simulink model "tb_adc_5g_spi_sys"  (Simulink 7.0)
settings: Solver=ode45  StartTime=0.0  StopTime=2000  RelTol=1e-3
libraries: xbsIndex_r4 x446, simulink x28, xps_library x12, dspsigops x12, xbsReplacements_r4 x4, casper_library x2
(part 1 of 5)
settings Model: Creator=user  LastModifiedBy=homin
settings DebuggingCC: SaveWithParameterizedLinksMsg=none

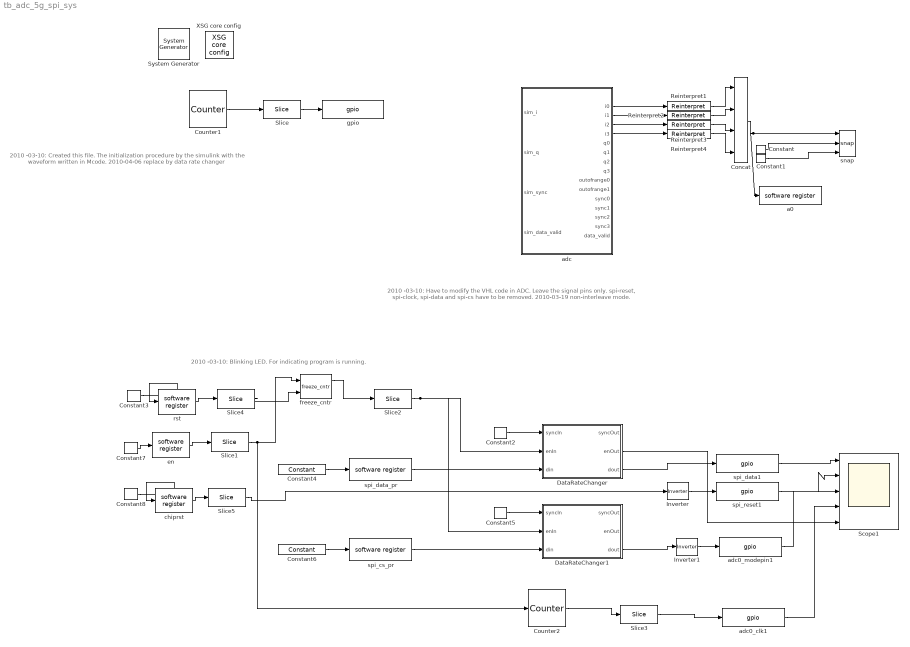
== system tb_adc_5g_spi_sys ==
  note: 2010 -03-10:
      | Created this file. The initialization procedure by the simulink with
      | the waveform written in Mcode.
      | 2010-04-06
      | replace by data rate changer
  note: 2010 -03-10:
      | Blinking LED. For indicating program is running.
  note: 2010 -03-10:
      | Have to modify the VHL code in ADC. Leave the signal pins only. spi-reset,
      | spi-clock, spi-data and spi-cs have to be removed.
      | 2010-03-19
      | non-interleave mode.
  " System Generator" : xbsIndex_r4/ System Generator  Tag=genX  SystemSampleTime=-1  xilinxfamily=virtex5  part=xc5vsx95t  speed=-1  package=ff1136  synthesis_tool=XST  clock_wrapper=Clock Enables  directory=./tb_adc_5g_spi_rw/sysgen  testbench=off  simulink_period=1  sysclk_period=5  dcm_input_clock_period=100  incr_netlist=off  trim_vbits=Everywhere in SubSystem  dbl_ovrd=According to Block Masks  core_generation=According to Block Masks  run_coregen=off  deprecated_control=off  eval_field=0  block_type=sysgen
      settings: block_version=10.1.3
  Concat : xbsIndex_r4/Concat  num_inputs=4  dbl_ovrd=off  block_type=concat
      settings: block_version=10.1.3
  Constant : xbsIndex_r4/Constant  arith_type=Boolean  const=0  n_bits=16  bin_pt=14  explicit_period=on  period=1  equ=P=C  opselect=C  inp2=PCIN>>17  opr=+  inp1=P  carry=CIN  dbl_ovrd=off  block_type=constant
  Constant1 : xbsIndex_r4/Constant  arith_type=Boolean  const=0  n_bits=16  bin_pt=14  explicit_period=on  period=1  equ=P=C  opselect=C  inp2=PCIN>>17  opr=+  inp1=P  carry=CIN  dbl_ovrd=off  block_type=constant
  Constant2 : xbsIndex_r4/Constant  arith_type=Boolean  const=1  n_bits=16  bin_pt=14  explicit_period=off  period=1  equ=P=C  opselect=C  inp2=PCIN>>17  opr=+  inp1=P  carry=CIN  dbl_ovrd=off  block_type=constant
  Constant3 : xbsIndex_r4/Constant  arith_type=Unsigned  const=0  n_bits=16  bin_pt=14  explicit_period=off  period=1  equ=P=C  opselect=C  inp2=PCIN>>17  opr=+  inp1=P  carry=CIN  dbl_ovrd=off  block_type=constant
  Constant4 : xbsIndex_r4/Constant  arith_type=Unsigned  const=8454984  n_bits=32  bin_pt=0  explicit_period=on  period=1  equ=P=C  opselect=C  inp2=PCIN>>17  opr=+  inp1=P  carry=CIN  dbl_ovrd=off  block_type=constant
  Constant5 : xbsIndex_r4/Constant  arith_type=Boolean  const=1  n_bits=16  bin_pt=14  explicit_period=off  period=1  equ=P=C  opselect=C  inp2=PCIN>>17  opr=+  inp1=P  carry=CIN  dbl_ovrd=off  block_type=constant
  Constant6 : xbsIndex_r4/Constant  arith_type=Unsigned  const=2^24 -1  n_bits=32  bin_pt=0  explicit_period=on  period=1  equ=P=C  opselect=C  inp2=PCIN>>17  opr=+  inp1=P  carry=CIN  dbl_ovrd=off  block_type=constant
  Constant7 : xbsIndex_r4/Constant  arith_type=Unsigned  const=1  n_bits=16  bin_pt=14  explicit_period=off  period=1  equ=P=C  opselect=C  inp2=PCIN>>17  opr=+  inp1=P  carry=CIN  dbl_ovrd=off  block_type=constant
  Constant8 : xbsIndex_r4/Constant  arith_type=Unsigned  const=0  n_bits=16  bin_pt=14  explicit_period=off  period=1  equ=P=C  opselect=C  inp2=PCIN>>17  opr=+  inp1=P  carry=CIN  dbl_ovrd=off  block_type=constant
  Counter1 : xbsIndex_r4/Counter  cnt_type=Free Running  cnt_to=Inf  operation=Up  start_count=0  cnt_by_val=1  arith_type=Unsigned  n_bits=27  bin_pt=0  load_pin=off  rst=off  en=off  explicit_period=on  period=1  dbl_ovrd=off  use_behavioral_HDL=off  use_rpm=off  implementation=Fabric  block_type=counter
  Counter2 : xbsIndex_r4/Counter  cnt_type=Free Running  cnt_to=8  operation=Up  start_count=0  cnt_by_val=1  arith_type=Unsigned  n_bits=4  bin_pt=0  load_pin=off  rst=off  en=on  explicit_period=on  period=1  dbl_ovrd=off  use_behavioral_HDL=off  use_rpm=off  implementation=Fabric  block_type=counter
  DataRateChanger : Subsystem  AncestorBlock=gavrt_library/DataRateChanger  mask(dataratechanger){input_length=1, ninputs=5, out_rate=4, in_bit_width=1, in_bin_pt=0, arith_type=0}
      mask prompts: input_length "Input Length (2^?)"; ninputs "Number of Simultaneous Inputs (2^?)"; out_rate "Output Rate (2^-?)"; in_bit_width "Input Bit Width"; in_bin_pt "Input Binary Point"; arith_type "Arithmetic Type (0=Unsigned, 1=Signed)"
      mask help:
      | Stores input data into a FIFO and then outputs the data at the specified data rate, cycling through inputs.
      | Thus if the input data looks like:
      | x0 x1 x2 x3 ...
      | y0 y1 y2 y3 ...
      | And the output rate is 2^-1, the output will look like this:
      | x0 x0 y0 y0 x1 x1 y1 y1 x2 x2 y2 y2...
      | enIn (enable In) should be high for 2^Input length clocks while the input data is valid.
      | *Currently enIn must be high in one burst of 2^Input length*
      | din should be all simultaneous inputs "crammed" together
      | enOut will be high for 2^(Input Length + Output Rate + Number of Simultaneous Inputs)
      | Arithmetic type and binary precision is only used for "uncramming" the input data
      mask init:
      | dataratechanger_init(gcb, 'input_length', input_length,...
      |     'ninputs', ninputs, ...
      |     'out_rate', out_rate,...
      |     'in_bit_width', in_bit_width,...
      |     'in_bin_pt', in_bin_pt,...
      |     'arith_type',arith_type);
      settings: AttributesFormatString=inputs=32, bit_width=1, input length=2, output rate=2^-4
  DataRateChanger1 : Subsystem  AncestorBlock=gavrt_library/DataRateChanger  mask(dataratechanger){input_length=1, ninputs=5, out_rate=4, in_bit_width=1, in_bin_pt=0, arith_type=0}
      mask prompts: input_length "Input Length (2^?)"; ninputs "Number of Simultaneous Inputs (2^?)"; out_rate "Output Rate (2^-?)"; in_bit_width "Input Bit Width"; in_bin_pt "Input Binary Point"; arith_type "Arithmetic Type (0=Unsigned, 1=Signed)"
      mask help:
      | Stores input data into a FIFO and then outputs the data at the specified data rate, cycling through inputs.
      | Thus if the input data looks like:
      | x0 x1 x2 x3 ...
      | y0 y1 y2 y3 ...
      | And the output rate is 2^-1, the output will look like this:
      | x0 x0 y0 y0 x1 x1 y1 y1 x2 x2 y2 y2...
      | enIn (enable In) should be high for 2^Input length clocks while the input data is valid.
      | *Currently enIn must be high in one burst of 2^Input length*
      | din should be all simultaneous inputs "crammed" together
      | enOut will be high for 2^(Input Length + Output Rate + Number of Simultaneous Inputs)
      | Arithmetic type and binary precision is only used for "uncramming" the input data
      mask init: same as tb_adc_5g_spi_sys/DataRateChanger
      settings: AttributesFormatString=inputs=32, bit_width=1, input length=2, output rate=2^-4
  Inverter : xbsIndex_r4/Inverter  en=off  latency=0  dbl_ovrd=off  block_type=inv
  Inverter1 : xbsIndex_r4/Inverter  en=off  latency=0  dbl_ovrd=off  block_type=inv
  Reinterpret{1..4} (4 alike) : xbsIndex_r4/Reinterpret  force_arith_type=on  arith_type=Unsigned  force_bin_pt=on  bin_pt=0  block_type=reinterpret
      settings: infoedit="Changes signal type without altering the binary representation.   You can changed the signal between signed and unsigned, and relocate the binary point.<P><P>Hardware notes: In hardware this block costs nothing.<P><P>Example:  Suppose the input is 6 bits wide, signed, with 2 fractional bits, and the output is forced to unsigned with 0 fractional bits.  Then an input of -2.0 (1110.00 in binary 2's complement) becomes an output of 56 (111000 in binary)."  block_version=10.1.3
  Scope1 : Scope  NumInputPorts=5
      settings: TickLabels=on  YMin=-1~-1~-1~-1~-5  YMax=2~2~2~2~5
  Slice : xbsIndex_r4/Slice  nbits=1  boolean_output=on  mode=Lower Bit Location + Width  bit1=27  base1=MSB of Input  bit0=26  base0=LSB of Input  dbl_ovrd=off  block_type=slice
      settings: infoedit="Extracts a given range of bits from each input sample and presents it at the output.  The output type is ordinarily unsigned with binary point at zero, but can be Boolean when the slice is one bit wide.<P><P>Hardware notes: In hardware this block costs nothing."  block_version=10.1.3
  Slice1 : xbsIndex_r4/Slice  nbits=1  boolean_output=on  mode=Lower Bit Location + Width  bit1=27  base1=MSB of Input  bit0=0  base0=LSB of Input  dbl_ovrd=off  block_type=slice
      settings: infoedit="Extracts a given range of bits from each input sample and presents it at the output.  The output type is ordinarily unsigned with binary point at zero, but can be Boolean when the slice is one bit wide.<P><P>Hardware notes: In hardware this block costs nothing."  block_version=10.1.3
  Slice2 : xbsIndex_r4/Slice  nbits=1  boolean_output=on  mode=Lower Bit Location + Width  bit1=27  base1=MSB of Input  bit0=4  base0=LSB of Input  dbl_ovrd=off  block_type=slice
      settings: infoedit="Extracts a given range of bits from each input sample and presents it at the output.  The output type is ordinarily unsigned with binary point at zero, but can be Boolean when the slice is one bit wide.<P><P>Hardware notes: In hardware this block costs nothing."  block_version=10.1.3
  Slice3 : xbsIndex_r4/Slice  nbits=1  boolean_output=on  mode=Lower Bit Location + Width  bit1=27  base1=MSB of Input  bit0=3  base0=LSB of Input  dbl_ovrd=off  block_type=slice
      settings: infoedit="Extracts a given range of bits from each input sample and presents it at the output.  The output type is ordinarily unsigned with binary point at zero, but can be Boolean when the slice is one bit wide.<P><P>Hardware notes: In hardware this block costs nothing."  block_version=10.1.3
  Slice4 : xbsIndex_r4/Slice  nbits=1  boolean_output=on  mode=Lower Bit Location + Width  bit1=27  base1=MSB of Input  bit0=0  base0=LSB of Input  dbl_ovrd=off  block_type=slice
      settings: infoedit="Extracts a given range of bits from each input sample and presents it at the output.  The output type is ordinarily unsigned with binary point at zero, but can be Boolean when the slice is one bit wide.<P><P>Hardware notes: In hardware this block costs nothing."  block_version=10.1.3
  Slice5 : xbsIndex_r4/Slice  nbits=1  boolean_output=on  mode=Lower Bit Location + Width  bit1=27  base1=MSB of Input  bit0=0  base0=LSB of Input  dbl_ovrd=off  block_type=slice
      settings: infoedit="Extracts a given range of bits from each input sample and presents it at the output.  The output type is ordinarily unsigned with binary point at zero, but can be Boolean when the slice is one bit wide.<P><P>Hardware notes: In hardware this block costs nothing."  block_version=10.1.3
  XSG core config : xps_library/XSG core config  Tag=xps:xsg  SystemSampleTime=-1  hw_sys=ROACH:sx95t  ibob_linux=off  clk_src=adc0_clk  iBOB_clk_src=sys_clk  BEE2_ctrl_clk_src=sys_clk  BEE2_usr_clk_src=sys_clk  ROACH_clk_src=adc0_clk  CORR_clk_src=sys_clk  gpio_clk_io_group=iBOB:sma  gpio_clk_bit_index=0  clk_rate=200  sample_period=1  synthesis_tool=XST  mpc_type=powerpc440_ext
  a0 : xps_library/software register  Tag=xps:sw_reg  SystemSampleTime=-1  io_dir=To Processor  arith_type=Unsigned  bitwidth=32  bin_pt=0  sample_period=1  gw_name=tb_adc_5g_spi_rw_a0_user_data_in
      link override convert: arith_type=Unsigned  n_bits=32  bin_pt=0
  adc : Subsystem  Tag=xps:adc_5g  mask(adc){adc_brd=adc0, adc_clk_rate=800, adc_interleave=off, sample_period=1}
      mask prompts: adc_brd "ADC board"; adc_clk_rate "ADC clock rate (MHz)"; adc_interleave "ADC interleave mode"; sample_period "Sample period"
      mask help: The ADC block converts analog inputs to digital outputs. Every clock cycle, the inputs are sampled and digitized to 8 bit binary point numbers in the range of [-1, 1) and are then output by the adc.
      mask init:
      | adc_5g_mask;
      mask Help: eval('xlWeb([getenv(''MLIB_ROOT''), ''\doc\html\sys_adc\sys_adc.html''])')
      mask StyleString: popup(adc0|adc1),edit,checkbox,edit
  adc0_clk1 : xps_library/gpio  Tag=xps:gpio  SystemSampleTime=-1  io_group=ROACH:zdok0  io_dir=out  arith_type=Boolean  bitwidth=1  bin_pt=0  bit_index=17  sample_period=1  use_single_ended=on  use_ddr=off  reg_iob=on  reg_clk_phase=0  termination=None
      link override convert: arith_type=Boolean  n_bits=1  bin_pt=0
  adc0_modepin1 : xps_library/gpio  Tag=xps:gpio  SystemSampleTime=-1  io_group=ROACH:zdok0  io_dir=out  arith_type=Boolean  bitwidth=1  bin_pt=0  bit_index=16  sample_period=1  use_single_ended=on  use_ddr=off  reg_iob=on  reg_clk_phase=0  termination=Pullup
      link override convert: arith_type=Boolean  n_bits=1  bin_pt=0
  chiprst : xps_library/software register  Tag=xps:sw_reg  SystemSampleTime=-1  io_dir=From Processor  arith_type=Unsigned  bitwidth=32  bin_pt=0  sample_period=1  gw_name=tb_adc_5g_spi_rw_chiprst_user_data_out
      link override convert: arith_type=Unsigned  n_bits=32  bin_pt=0
      link override sandbox_spi_cs_pr_user_data_out: arith_type=Unsigned  n_bits=32  bin_pt=0  period=1
      link override sandbox_spi_data_pr_user_data_out: arith_type=Unsigned  n_bits=32  bin_pt=0  period=1
      link override spi_rw_en_user_data_out: arith_type=Unsigned  n_bits=32  bin_pt=0  period=1
      link override spi_rw_rst_user_data_out: arith_type=Unsigned  n_bits=32  bin_pt=0  period=1
      link override spi_rw_spi_data_pr_user_data_out: arith_type=Unsigned  n_bits=32  bin_pt=0  period=1
      link override tb_adc_5g_gpioADCclk_rst_user_data_out: arith_type=Unsigned  n_bits=32  bin_pt=0  period=1
      link override tb_adc_5g_spi_rw_chiprst_user_data_out: arith_type=Unsigned  n_bits=32  bin_pt=0  period=1
      link override tb_adc_5g_spi_rw_rst_user_data_out: arith_type=Unsigned  n_bits=32  bin_pt=0  period=1
  en : xps_library/software register  Tag=xps:sw_reg  SystemSampleTime=-1  io_dir=From Processor  arith_type=Unsigned  bitwidth=32  bin_pt=0  sample_period=1  gw_name=tb_adc_5g_spi_rw_en_user_data_out
      link override convert: arith_type=Unsigned  n_bits=32  bin_pt=0
      link override sandbox_spi_cs_pr_user_data_out: arith_type=Unsigned  n_bits=32  bin_pt=0  period=1
      link override sandbox_spi_data_pr_user_data_out: arith_type=Unsigned  n_bits=32  bin_pt=0  period=1
      link override spi_rw_en_user_data_out: arith_type=Unsigned  n_bits=32  bin_pt=0  period=1
      link override spi_rw_spi_data_pr_user_data_out: arith_type=Unsigned  n_bits=32  bin_pt=0  period=1
      link override tb_adc_5g_gpioADCclk_en_user_data_out: arith_type=Unsigned  n_bits=32  bin_pt=0  period=1
      link override tb_adc_5g_spi_rw_en_user_data_out: arith_type=Unsigned  n_bits=32  bin_pt=0  period=1
  freeze_cntr : casper_library/Misc/freeze_cntr  SystemSampleTime=-1  CounterBits=5
  gpio : xps_library/gpio  Tag=xps:gpio  SystemSampleTime=-1  io_group=ROACH:led  io_dir=out  arith_type=Boolean  bitwidth=1  bin_pt=0  bit_index=1  sample_period=1  use_single_ended=off  use_ddr=off  reg_iob=on  reg_clk_phase=0  termination=None
      link override convert: arith_type=Boolean  n_bits=1  bin_pt=0
  rst : xps_library/software register  Tag=xps:sw_reg  SystemSampleTime=-1  io_dir=From Processor  arith_type=Unsigned  bitwidth=32  bin_pt=0  sample_period=1  gw_name=tb_adc_5g_spi_rw_rst_user_data_out
      link override convert: arith_type=Unsigned  n_bits=32  bin_pt=0
      link override sandbox_spi_cs_pr_user_data_out: arith_type=Unsigned  n_bits=32  bin_pt=0  period=1
      link override sandbox_spi_data_pr_user_data_out: arith_type=Unsigned  n_bits=32  bin_pt=0  period=1
      link override spi_rw_en_user_data_out: arith_type=Unsigned  n_bits=32  bin_pt=0  period=1
      link override spi_rw_rst_user_data_out: arith_type=Unsigned  n_bits=32  bin_pt=0  period=1
      link override spi_rw_spi_data_pr_user_data_out: arith_type=Unsigned  n_bits=32  bin_pt=0  period=1
      link override tb_adc_5g_gpioADCclk_rst_user_data_out: arith_type=Unsigned  n_bits=32  bin_pt=0  period=1
      link override tb_adc_5g_spi_rw_rst_user_data_out: arith_type=Unsigned  n_bits=32  bin_pt=0  period=1
  snap : casper_library/Scopes/snap  SystemSampleTime=-1  nsamples=11
      link override addr/convert: arith_type=Unsigned  n_bits=32  bin_pt=0
      link override bram/convert_din: arith_type=Unsigned
      link override bram/mem/sim_data_in: arith_type=Unsigned
      link override bram/tb_adc_5g_gpioADCclk_snap_bram_data_out: arith_type=Unsigned
      link override bram/tb_adc_5g_spi_rw_snap_bram_data_out: arith_type=Unsigned
      link override bram/tb_adc_5g_sysclk_snap_bram_data_out: arith_type=Unsigned
      link override ctrl/tb_adc_5g_gpioADCclk_snap_ctrl_user_data_out: arith_type=Unsigned  n_bits=32  bin_pt=0  period=1
      link override ctrl/tb_adc_5g_spi_rw_snap_ctrl_user_data_out: arith_type=Unsigned  n_bits=32  bin_pt=0  period=1
      link override ctrl/tb_adc_5g_sysclk_snap_ctrl_user_data_out: arith_type=Unsigned  n_bits=32  bin_pt=0  period=1
  spi_cs_pr : xps_library/software register  Tag=xps:sw_reg  SystemSampleTime=-1  io_dir=From Processor  arith_type=Unsigned  bitwidth=32  bin_pt=0  sample_period=1  gw_name=tb_adc_5g_spi_rw_spi_cs_pr_user_data_out
      link override convert: arith_type=Unsigned  n_bits=32  bin_pt=0
      link override sandbox_spi_cs_pr_user_data_out: arith_type=Unsigned  n_bits=32  bin_pt=0  period=1
      link override spi_rw_spi_cs_pr_user_data_out: arith_type=Unsigned  n_bits=32  bin_pt=0  period=1
      link override tb_adc_5g_gpioADCclk_spi_cs_pr_user_data_out: arith_type=Unsigned  n_bits=32  bin_pt=0  period=1
      link override tb_adc_5g_spi_rw_spi_cs_pr_user_data_out: arith_type=Unsigned  n_bits=32  bin_pt=0  period=1
  spi_data1 : xps_library/gpio  Tag=xps:gpio  SystemSampleTime=-1  io_group=ROACH:zdok0  io_dir=out  arith_type=Boolean  bitwidth=1  bin_pt=0  bit_index=18  sample_period=1  use_single_ended=on  use_ddr=off  reg_iob=on  reg_clk_phase=0  termination=None
      link override convert: arith_type=Boolean  n_bits=1  bin_pt=0
  spi_data_pr : xps_library/software register  Tag=xps:sw_reg  SystemSampleTime=-1  io_dir=From Processor  arith_type=Unsigned  bitwidth=32  bin_pt=0  sample_period=1  gw_name=tb_adc_5g_spi_rw_spi_data_pr_user_data_out
      link override convert: arith_type=Unsigned  n_bits=32  bin_pt=0
      link override sandbox_spi_cs_pr_user_data_out: arith_type=Unsigned  n_bits=32  bin_pt=0  period=1
      link override sandbox_spi_data_pr_user_data_out: arith_type=Unsigned  n_bits=32  bin_pt=0  period=1
      link override spi_rw_spi_data_pr_user_data_out: arith_type=Unsigned  n_bits=32  bin_pt=0  period=1
      link override tb_adc_5g_gpioADCclk_spi_data_pr_user_data_out: arith_type=Unsigned  n_bits=32  bin_pt=0  period=1
      link override tb_adc_5g_spi_rw_spi_data_pr_user_data_out: arith_type=Unsigned  n_bits=32  bin_pt=0  period=1
  spi_reset1 : xps_library/gpio  Tag=xps:gpio  SystemSampleTime=-1  io_group=ROACH:zdok0  io_dir=out  arith_type=Boolean  bitwidth=1  bin_pt=0  bit_index=36  sample_period=1  use_single_ended=on  use_ddr=off  reg_iob=on  reg_clk_phase=0  termination=Pullup
      link override convert: arith_type=Boolean  n_bits=1  bin_pt=0
  wires:
  Counter1/1 -> Slice/1
  Slice/1 -> gpio/1
  Reinterpret1/1 -> Concat/1
  Reinterpret2/1 -> Concat/2
  Reinterpret3/1 -> Concat/3
  Reinterpret4/1 -> Concat/4
  Concat/1 -> snap/1, a0/1
  Constant/1 -> snap/2
  Constant1/1 -> snap/3
  adc/1(i0) -> Reinterpret1/1
  adc/2(i1) -> Reinterpret2/1
  adc/3(i2) -> Reinterpret3/1
  adc/4(i3) -> Reinterpret4/1
  spi_data1/1 -> Scope1/1
  spi_data_pr/1 -> DataRateChanger/3(din)
  Constant4/1 -> spi_data_pr/1
  Slice2/1 -> DataRateChanger1/2(enIn), DataRateChanger/2(enIn)
  Constant2/1 -> DataRateChanger/1(syncIn)
  DataRateChanger/3(dout) -> spi_data1/1
  adc0_clk1/1 -> Scope1/4
  Counter2/1 -> Slice3/1
  Slice3/1 -> adc0_clk1/1
  Slice1/1 -> freeze_cntr/1, Counter2/1
  freeze_cntr/1 -> Slice2/1
  Slice4/1 -> freeze_cntr/2
  adc0_modepin1/1 -> Scope1/3
  spi_cs_pr/1 -> DataRateChanger1/3(din)
  Constant6/1 -> spi_cs_pr/1
  Constant5/1 -> DataRateChanger1/1(syncIn)
  DataRateChanger1/3(dout) -> Inverter1/1
  DataRateChanger/2(enOut) -> Scope1/5
  spi_reset1/1 -> Scope1/2
  en/1 -> Slice1/1
  rst/1 -> Slice4/1
  Constant3/1 -> rst/1
  Constant7/1 -> en/1
  Inverter/1 -> spi_reset1/1
  Inverter1/1 -> adc0_modepin1/1
  Slice5/1 -> Inverter/1
  chiprst/1 -> Slice5/1
  Constant8/1 -> chiprst/1

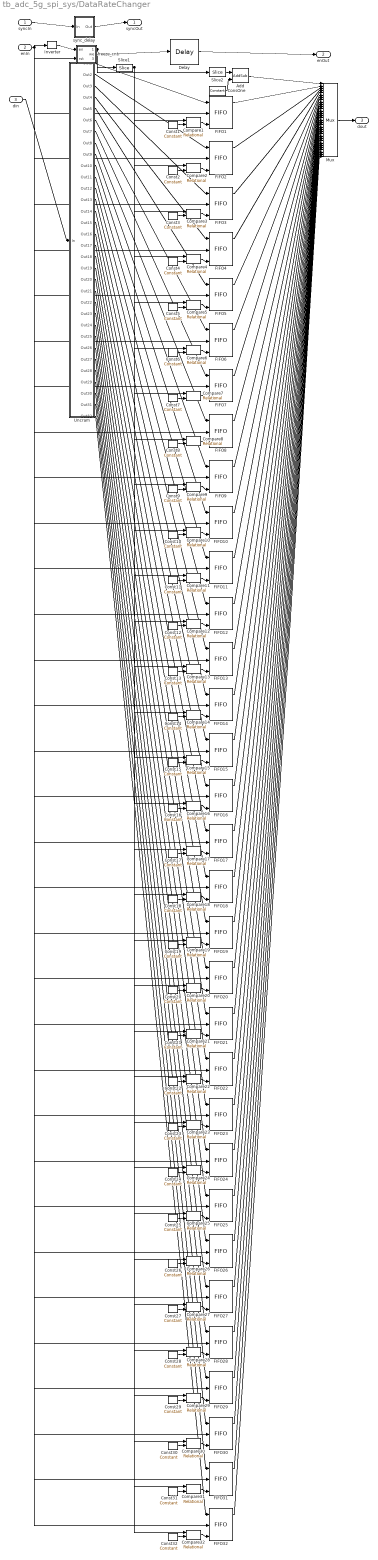
== system tb_adc_5g_spi_sys/DataRateChanger ==
  syncIn : Inport  OutDataType=sfix(16)  OutScaling=2^0
  enIn : Inport  Port=2  OutDataType=sfix(16)  OutScaling=2^0
  din : Inport  Port=3  OutDataType=sfix(16)  OutScaling=2^0
  Add : xbsIndex_r4/AddSub  mode=Addition  use_carryin=off  use_carryout=off  en=off  latency=0  precision=User Defined  arith_type=Unsigned  n_bits=5  bin_pt=0  quantization=Truncate  overflow=Wrap  dbl_ovrd=off  use_behavioral_HDL=off  pipelined=off  use_rpm=on  hw_selection=Fabric  block_type=addsub
      settings: block_version=10.1.3
  Compare{1..32} (32 alike) : xbsIndex_r4/Relational  mode=a=b  en=off  latency=0  dbl_ovrd=off  block_type=relational
      Compare1 settings: xl_area=[0, 0, 0, 0, 0, 0, 0]  block_version=10.1.2
      Compare10 settings: block_version=10.1.3
      Compare11 settings: block_version=10.1.3
      Compare12 settings: block_version=10.1.3
      Compare13 settings: block_version=10.1.3
      Compare14 settings: block_version=10.1.3
      Compare15 settings: block_version=10.1.3
      Compare16 settings: block_version=10.1.3
      Compare17 settings: block_version=10.1.3
      Compare18 settings: block_version=10.1.3
      Compare19 settings: block_version=10.1.3
      Compare2 settings: block_version=10.1.3
      Compare20 settings: block_version=10.1.3
      Compare21 settings: block_version=10.1.3
      Compare22 settings: block_version=10.1.3
      Compare23 settings: block_version=10.1.3
      Compare24 settings: block_version=10.1.3
      Compare25 settings: block_version=10.1.3
      Compare26 settings: block_version=10.1.3
      Compare27 settings: block_version=10.1.3
      Compare28 settings: block_version=10.1.3
      Compare29 settings: block_version=10.1.3
      Compare3 settings: block_version=10.1.3
      Compare30 settings: block_version=10.1.3
      Compare31 settings: block_version=10.1.3
      Compare32 settings: block_version=10.1.3
      Compare4 settings: block_version=10.1.3
      Compare5 settings: block_version=10.1.3
      Compare6 settings: block_version=10.1.3
      Compare7 settings: block_version=10.1.3
      Compare8 settings: block_version=10.1.3
      Compare9 settings: block_version=10.1.3
  ConsOne : xbsIndex_r4/Constant  arith_type=Unsigned  const=1  n_bits=1  bin_pt=0  explicit_period=off  period=1  equ=P=C  opselect=C  inp2=PCIN>>17  opr=+  inp1=P  carry=CIN  dbl_ovrd=off  block_type=constant
  Const1 : xbsIndex_r4/Constant  arith_type=Unsigned  const=1  n_bits=9  bin_pt=0  explicit_period=off  period=1  equ=P=C  opselect=C  inp2=PCIN>>17  opr=+  inp1=P  carry=CIN  dbl_ovrd=off  block_type=constant
      settings: block_version=10.1.2
  Const10 : xbsIndex_r4/Constant  arith_type=Unsigned  const=145  n_bits=9  bin_pt=0  explicit_period=off  period=1  equ=P=C  opselect=C  inp2=PCIN>>17  opr=+  inp1=P  carry=CIN  dbl_ovrd=off  block_type=constant
  Const11 : xbsIndex_r4/Constant  arith_type=Unsigned  const=161  n_bits=9  bin_pt=0  explicit_period=off  period=1  equ=P=C  opselect=C  inp2=PCIN>>17  opr=+  inp1=P  carry=CIN  dbl_ovrd=off  block_type=constant
  Const12 : xbsIndex_r4/Constant  arith_type=Unsigned  const=177  n_bits=9  bin_pt=0  explicit_period=off  period=1  equ=P=C  opselect=C  inp2=PCIN>>17  opr=+  inp1=P  carry=CIN  dbl_ovrd=off  block_type=constant
  Const13 : xbsIndex_r4/Constant  arith_type=Unsigned  const=193  n_bits=9  bin_pt=0  explicit_period=off  period=1  equ=P=C  opselect=C  inp2=PCIN>>17  opr=+  inp1=P  carry=CIN  dbl_ovrd=off  block_type=constant
  Const14 : xbsIndex_r4/Constant  arith_type=Unsigned  const=209  n_bits=9  bin_pt=0  explicit_period=off  period=1  equ=P=C  opselect=C  inp2=PCIN>>17  opr=+  inp1=P  carry=CIN  dbl_ovrd=off  block_type=constant
  Const15 : xbsIndex_r4/Constant  arith_type=Unsigned  const=225  n_bits=9  bin_pt=0  explicit_period=off  period=1  equ=P=C  opselect=C  inp2=PCIN>>17  opr=+  inp1=P  carry=CIN  dbl_ovrd=off  block_type=constant
  Const16 : xbsIndex_r4/Constant  arith_type=Unsigned  const=241  n_bits=9  bin_pt=0  explicit_period=off  period=1  equ=P=C  opselect=C  inp2=PCIN>>17  opr=+  inp1=P  carry=CIN  dbl_ovrd=off  block_type=constant
  Const17 : xbsIndex_r4/Constant  arith_type=Unsigned  const=257  n_bits=9  bin_pt=0  explicit_period=off  period=1  equ=P=C  opselect=C  inp2=PCIN>>17  opr=+  inp1=P  carry=CIN  dbl_ovrd=off  block_type=constant
  Const18 : xbsIndex_r4/Constant  arith_type=Unsigned  const=273  n_bits=9  bin_pt=0  explicit_period=off  period=1  equ=P=C  opselect=C  inp2=PCIN>>17  opr=+  inp1=P  carry=CIN  dbl_ovrd=off  block_type=constant
  Const19 : xbsIndex_r4/Constant  arith_type=Unsigned  const=289  n_bits=9  bin_pt=0  explicit_period=off  period=1  equ=P=C  opselect=C  inp2=PCIN>>17  opr=+  inp1=P  carry=CIN  dbl_ovrd=off  block_type=constant
  Const2 : xbsIndex_r4/Constant  arith_type=Unsigned  const=17  n_bits=9  bin_pt=0  explicit_period=off  period=1  equ=P=C  opselect=C  inp2=PCIN>>17  opr=+  inp1=P  carry=CIN  dbl_ovrd=off  block_type=constant
  Const20 : xbsIndex_r4/Constant  arith_type=Unsigned  const=305  n_bits=9  bin_pt=0  explicit_period=off  period=1  equ=P=C  opselect=C  inp2=PCIN>>17  opr=+  inp1=P  carry=CIN  dbl_ovrd=off  block_type=constant
  Const21 : xbsIndex_r4/Constant  arith_type=Unsigned  const=321  n_bits=9  bin_pt=0  explicit_period=off  period=1  equ=P=C  opselect=C  inp2=PCIN>>17  opr=+  inp1=P  carry=CIN  dbl_ovrd=off  block_type=constant
  Const22 : xbsIndex_r4/Constant  arith_type=Unsigned  const=337  n_bits=9  bin_pt=0  explicit_period=off  period=1  equ=P=C  opselect=C  inp2=PCIN>>17  opr=+  inp1=P  carry=CIN  dbl_ovrd=off  block_type=constant
  Const23 : xbsIndex_r4/Constant  arith_type=Unsigned  const=353  n_bits=9  bin_pt=0  explicit_period=off  period=1  equ=P=C  opselect=C  inp2=PCIN>>17  opr=+  inp1=P  carry=CIN  dbl_ovrd=off  block_type=constant
  Const24 : xbsIndex_r4/Constant  arith_type=Unsigned  const=369  n_bits=9  bin_pt=0  explicit_period=off  period=1  equ=P=C  opselect=C  inp2=PCIN>>17  opr=+  inp1=P  carry=CIN  dbl_ovrd=off  block_type=constant
  Const25 : xbsIndex_r4/Constant  arith_type=Unsigned  const=385  n_bits=9  bin_pt=0  explicit_period=off  period=1  equ=P=C  opselect=C  inp2=PCIN>>17  opr=+  inp1=P  carry=CIN  dbl_ovrd=off  block_type=constant
  Const26 : xbsIndex_r4/Constant  arith_type=Unsigned  const=401  n_bits=9  bin_pt=0  explicit_period=off  period=1  equ=P=C  opselect=C  inp2=PCIN>>17  opr=+  inp1=P  carry=CIN  dbl_ovrd=off  block_type=constant
  Const27 : xbsIndex_r4/Constant  arith_type=Unsigned  const=417  n_bits=9  bin_pt=0  explicit_period=off  period=1  equ=P=C  opselect=C  inp2=PCIN>>17  opr=+  inp1=P  carry=CIN  dbl_ovrd=off  block_type=constant
  Const28 : xbsIndex_r4/Constant  arith_type=Unsigned  const=433  n_bits=9  bin_pt=0  explicit_period=off  period=1  equ=P=C  opselect=C  inp2=PCIN>>17  opr=+  inp1=P  carry=CIN  dbl_ovrd=off  block_type=constant
  Const29 : xbsIndex_r4/Constant  arith_type=Unsigned  const=449  n_bits=9  bin_pt=0  explicit_period=off  period=1  equ=P=C  opselect=C  inp2=PCIN>>17  opr=+  inp1=P  carry=CIN  dbl_ovrd=off  block_type=constant
  Const3 : xbsIndex_r4/Constant  arith_type=Unsigned  const=33  n_bits=9  bin_pt=0  explicit_period=off  period=1  equ=P=C  opselect=C  inp2=PCIN>>17  opr=+  inp1=P  carry=CIN  dbl_ovrd=off  block_type=constant
  Const30 : xbsIndex_r4/Constant  arith_type=Unsigned  const=465  n_bits=9  bin_pt=0  explicit_period=off  period=1  equ=P=C  opselect=C  inp2=PCIN>>17  opr=+  inp1=P  carry=CIN  dbl_ovrd=off  block_type=constant
  Const31 : xbsIndex_r4/Constant  arith_type=Unsigned  const=481  n_bits=9  bin_pt=0  explicit_period=off  period=1  equ=P=C  opselect=C  inp2=PCIN>>17  opr=+  inp1=P  carry=CIN  dbl_ovrd=off  block_type=constant
  Const32 : xbsIndex_r4/Constant  arith_type=Unsigned  const=497  n_bits=9  bin_pt=0  explicit_period=off  period=1  equ=P=C  opselect=C  inp2=PCIN>>17  opr=+  inp1=P  carry=CIN  dbl_ovrd=off  block_type=constant
  Const4 : xbsIndex_r4/Constant  arith_type=Unsigned  const=49  n_bits=9  bin_pt=0  explicit_period=off  period=1  equ=P=C  opselect=C  inp2=PCIN>>17  opr=+  inp1=P  carry=CIN  dbl_ovrd=off  block_type=constant
  Const5 : xbsIndex_r4/Constant  arith_type=Unsigned  const=65  n_bits=9  bin_pt=0  explicit_period=off  period=1  equ=P=C  opselect=C  inp2=PCIN>>17  opr=+  inp1=P  carry=CIN  dbl_ovrd=off  block_type=constant
  Const6 : xbsIndex_r4/Constant  arith_type=Unsigned  const=81  n_bits=9  bin_pt=0  explicit_period=off  period=1  equ=P=C  opselect=C  inp2=PCIN>>17  opr=+  inp1=P  carry=CIN  dbl_ovrd=off  block_type=constant
  Const7 : xbsIndex_r4/Constant  arith_type=Unsigned  const=97  n_bits=9  bin_pt=0  explicit_period=off  period=1  equ=P=C  opselect=C  inp2=PCIN>>17  opr=+  inp1=P  carry=CIN  dbl_ovrd=off  block_type=constant
  Const8 : xbsIndex_r4/Constant  arith_type=Unsigned  const=113  n_bits=9  bin_pt=0  explicit_period=off  period=1  equ=P=C  opselect=C  inp2=PCIN>>17  opr=+  inp1=P  carry=CIN  dbl_ovrd=off  block_type=constant
  Const9 : xbsIndex_r4/Constant  arith_type=Unsigned  const=129  n_bits=9  bin_pt=0  explicit_period=off  period=1  equ=P=C  opselect=C  inp2=PCIN>>17  opr=+  inp1=P  carry=CIN  dbl_ovrd=off  block_type=constant
  Delay : xbsIndex_r4/Delay  en=off  latency=3  dbl_ovrd=off  reg_retiming=off  block_type=delay
      settings: block_version=10.1.2
  FIFO1 : xbsIndex_r4/FIFO  depth=16  percent_nbits=1  rst=off  en=off  use_dcount=off  use_almost_empty=off  almost_empty_thresh=2  use_almost_full=off  almost_full_thresh=14  dbl_ovrd=off  mem_type=Block RAM  explicit_period=off  period=1  block_type=fifo
      settings: xl_area=[0, 0, 0, 0, 0, 0, 0]  block_version=10.1.2
  FIFO{2..32} (31 alike) : xbsIndex_r4/FIFO  depth=16  percent_nbits=1  rst=off  en=off  use_dcount=off  use_almost_empty=off  almost_empty_thresh=2  use_almost_full=off  almost_full_thresh=14  dbl_ovrd=off  mem_type=Block RAM  block_type=fifo
      settings: block_version=10.1.3
  Inverter : xbsIndex_r4/Inverter  en=off  latency=0  dbl_ovrd=off  block_type=inv
      settings: xl_area=[0, 0, 0, 0, 0, 0, 0]  block_version=10.1.2
  Mux : xbsIndex_r4/Mux  inputs=32  en=off  latency=1  precision=Full  arith_type=Unsigned  n_bits=16  bin_pt=14  quantization=Truncate  overflow=Wrap  dbl_ovrd=off  block_type=mux
  Slice1 : xbsIndex_r4/Slice  nbits=9  boolean_output=off  mode=Lower Bit Location + Width  bit1=0  base1=MSB of Input  bit0=0  base0=LSB of Input  dbl_ovrd=off  block_type=slice
      settings: infoedit="Extracts a given range of bits from each input sample and presents it at the output.  The output type is ordinarily unsigned with binary point at zero, but can be Boolean when the slice is one bit wide.<P><P>Hardware notes: In hardware this block costs nothing."  block_version=10.1.2
  Slice2 : xbsIndex_r4/Slice  nbits=5  boolean_output=off  mode=Lower Bit Location + Width  bit1=0  base1=MSB of Input  bit0=4  base0=LSB of Input  dbl_ovrd=off  block_type=slice
      settings: infoedit="Extracts a given range of bits from each input sample and presents it at the output.  The output type is ordinarily unsigned with binary point at zero, but can be Boolean when the slice is one bit wide.<P><P>Hardware notes: In hardware this block costs nothing."  block_version=10.1.3
  Uncram : Subsystem  AncestorBlock=gavrt_library/uncram  mask(uncram){num_slice=32, slice_width=1, bin_pt=0, arith_type=0}
      mask prompts: num_slice "Number of slices"; slice_width "Slice Width"; bin_pt "Output Binary Point"; arith_type "Output Arithmetic Type (0=Unsigned, 1=Signed)"
      mask help: Takes a concatenated input and slices it up into even pieces and reinterprets them as signed fixed point numbers with a given binary point.
      mask init:
      | uncram_init(gcb, ...
      |     'num_slice', num_slice, ...
      |     'slice_width', slice_width, ...
      |     'bin_pt', bin_pt, ...
      |     'arith_type', arith_type);
      settings: AttributesFormatString=UFix_1_0
  freeze_cntr : Subsystem  AncestorBlock=casper_library/Misc/freeze_cntr  mask(freeze_cntr){CounterBits=10}
      mask prompts: CounterBits "Counter Length (2^?)"
      mask help:
      | A freeze counter is an enabled counter which holds its final value (regardless of enables)
      | until it is reset.
      mask Help: eval('xlWeb([getenv(''MLIB_ROOT''), ''\casper_library\doc\freeze_cntr_usage.html''])')
  sync_delay : Subsystem  AncestorBlock=casper_library/Delays/sync_delay  mask(sync_delay){DelayLen=5}
      mask prompts: DelayLen "Delay Length:"
      mask help: Delay an infrequent boolean pulse by the specified number of clocks.
      mask init:
      | BitWidth = max(2, ceil(log2(DelayLen+1)));
      | UseCounter = 1;
      | if DelayLen == 0,
      | 	UseCounter = 0;
      | end
      mask Help: eval('xlWeb([getenv(''MLIB_ROOT''), ''\casper_library\doc\sync_delay_usage.html''])')
      mask Display: fprintf('Z^-%d', DelayLen)
  syncOut : Outport  OutDataType=sfix(16)  OutScaling=2^0
  enOut : Outport  Port=2  OutDataType=sfix(16)  OutScaling=2^0
  dout : Outport  Port=3  OutDataType=sfix(16)  OutScaling=2^0
  wires:
  syncIn/1 -> sync_delay/1(In)
  sync_delay/1(Out) -> syncOut/1
  enIn/1 -> Inverter/1, freeze_cntr/2(rst), FIFO1/2, FIFO2/2, FIFO3/2, FIFO4/2, FIFO5/2, FIFO6/2, FIFO7/2, FIFO8/2, FIFO9/2, FIFO10/2, FIFO11/2, FIFO12/2, FIFO13/2, FIFO14/2, FIFO15/2, FIFO16/2, FIFO17/2, FIFO18/2, FIFO19/2, FIFO20/2, FIFO21/2, FIFO22/2, FIFO23/2, FIFO24/2, FIFO25/2, FIFO26/2, FIFO27/2, FIFO28/2, FIFO29/2, FIFO30/2, FIFO31/2, FIFO32/2
  Inverter/1 -> freeze_cntr/1(en)
  freeze_cntr/2(we) -> Delay/1
  Delay/1 -> enOut/1
  freeze_cntr/1(addr) -> Slice1/1, Slice2/1
  din/1 -> Uncram/1(In)
  Mux/1 -> dout/1
  Slice2/1 -> Add/1
  ConsOne/1 -> Add/2
  Add/1 -> Mux/1
  Const1/1 -> Compare1/2
  Compare1/1 -> FIFO1/3
  Uncram/1(Out1) -> FIFO1/1
  FIFO1/1 -> Mux/2
  Slice1/1 -> Compare1/1, Compare2/1, Compare3/1, Compare4/1, Compare5/1, Compare6/1, Compare7/1, Compare8/1, Compare9/1, Compare10/1, Compare11/1, Compare12/1, Compare13/1, Compare14/1, Compare15/1, Compare16/1, Compare17/1, Compare18/1, Compare19/1, Compare20/1, Compare21/1, Compare22/1, Compare23/1, Compare24/1, Compare25/1, Compare26/1, Compare27/1, Compare28/1, Compare29/1, Compare30/1, Compare31/1, Compare32/1
  Const2/1 -> Compare2/2
  Compare2/1 -> FIFO2/3
  Uncram/2(Out2) -> FIFO2/1
  FIFO2/1 -> Mux/3
  Const3/1 -> Compare3/2
  Compare3/1 -> FIFO3/3
  Uncram/3(Out3) -> FIFO3/1
  FIFO3/1 -> Mux/4
  Const4/1 -> Compare4/2
  Compare4/1 -> FIFO4/3
  Uncram/4(Out4) -> FIFO4/1
  FIFO4/1 -> Mux/5
  Const5/1 -> Compare5/2
  Compare5/1 -> FIFO5/3
  Uncram/5(Out5) -> FIFO5/1
  FIFO5/1 -> Mux/6
  Const6/1 -> Compare6/2
  Compare6/1 -> FIFO6/3
  Uncram/6(Out6) -> FIFO6/1
  FIFO6/1 -> Mux/7
  Const7/1 -> Compare7/2
  Compare7/1 -> FIFO7/3
  Uncram/7(Out7) -> FIFO7/1
  FIFO7/1 -> Mux/8
  Const8/1 -> Compare8/2
  Compare8/1 -> FIFO8/3
  Uncram/8(Out8) -> FIFO8/1
  FIFO8/1 -> Mux/9
  Const9/1 -> Compare9/2
  Compare9/1 -> FIFO9/3
  Uncram/9(Out9) -> FIFO9/1
  FIFO9/1 -> Mux/10
  Const10/1 -> Compare10/2
  Compare10/1 -> FIFO10/3
  Uncram/10(Out10) -> FIFO10/1
  FIFO10/1 -> Mux/11
  Const11/1 -> Compare11/2
  Compare11/1 -> FIFO11/3
  Uncram/11(Out11) -> FIFO11/1
  FIFO11/1 -> Mux/12
  Const12/1 -> Compare12/2
  Compare12/1 -> FIFO12/3
  Uncram/12(Out12) -> FIFO12/1
  FIFO12/1 -> Mux/13
  Const13/1 -> Compare13/2
  Compare13/1 -> FIFO13/3
  Uncram/13(Out13) -> FIFO13/1
  FIFO13/1 -> Mux/14
  Const14/1 -> Compare14/2
  Compare14/1 -> FIFO14/3
  Uncram/14(Out14) -> FIFO14/1
  FIFO14/1 -> Mux/15
  Const15/1 -> Compare15/2
  Compare15/1 -> FIFO15/3
  Uncram/15(Out15) -> FIFO15/1
  FIFO15/1 -> Mux/16
  Const16/1 -> Compare16/2
  Compare16/1 -> FIFO16/3
  Uncram/16(Out16) -> FIFO16/1
  FIFO16/1 -> Mux/17
  Const17/1 -> Compare17/2
  Compare17/1 -> FIFO17/3
  Uncram/17(Out17) -> FIFO17/1
  FIFO17/1 -> Mux/18
  Const18/1 -> Compare18/2
  Compare18/1 -> FIFO18/3
  Uncram/18(Out18) -> FIFO18/1
  FIFO18/1 -> Mux/19
  Const19/1 -> Compare19/2
  Compare19/1 -> FIFO19/3
  Uncram/19(Out19) -> FIFO19/1
  FIFO19/1 -> Mux/20
  Const20/1 -> Compare20/2
  Compare20/1 -> FIFO20/3
  Uncram/20(Out20) -> FIFO20/1
  FIFO20/1 -> Mux/21
  Const21/1 -> Compare21/2
  Compare21/1 -> FIFO21/3
  Uncram/21(Out21) -> FIFO21/1
  FIFO21/1 -> Mux/22
  Const22/1 -> Compare22/2
  Compare22/1 -> FIFO22/3
  Uncram/22(Out22) -> FIFO22/1
  FIFO22/1 -> Mux/23
  Const23/1 -> Compare23/2
  Compare23/1 -> FIFO23/3
  Uncram/23(Out23) -> FIFO23/1
  FIFO23/1 -> Mux/24
  Const24/1 -> Compare24/2
  Compare24/1 -> FIFO24/3
  Uncram/24(Out24) -> FIFO24/1
  FIFO24/1 -> Mux/25
  Const25/1 -> Compare25/2
  Compare25/1 -> FIFO25/3
  Uncram/25(Out25) -> FIFO25/1
  FIFO25/1 -> Mux/26
  Const26/1 -> Compare26/2
  Compare26/1 -> FIFO26/3
  Uncram/26(Out26) -> FIFO26/1
  FIFO26/1 -> Mux/27
  Const27/1 -> Compare27/2
  Compare27/1 -> FIFO27/3
  Uncram/27(Out27) -> FIFO27/1
  FIFO27/1 -> Mux/28
  Const28/1 -> Compare28/2
  Compare28/1 -> FIFO28/3
  Uncram/28(Out28) -> FIFO28/1
  FIFO28/1 -> Mux/29
  Const29/1 -> Compare29/2
  Compare29/1 -> FIFO29/3
  Uncram/29(Out29) -> FIFO29/1
  FIFO29/1 -> Mux/30
  Const30/1 -> Compare30/2
  Compare30/1 -> FIFO30/3
  Uncram/30(Out30) -> FIFO30/1
  FIFO30/1 -> Mux/31
  Const31/1 -> Compare31/2
  Compare31/1 -> FIFO31/3
  Uncram/31(Out31) -> FIFO31/1
  FIFO31/1 -> Mux/32
  Const32/1 -> Compare32/2
  Compare32/1 -> FIFO32/3
  Uncram/32(Out32) -> FIFO32/1
  FIFO32/1 -> Mux/33
